simulink model "hexAddFm"  (R2024a)
settings: configuration reference "standardSILConfiguraitonParams" (kept outside this file)
settings Model: Creator=GTAR  LastModifiedBy=jerem
settings ConfigSetRef: SourceName=standardSILConfiguraitonParams  SourceLocation=Base Workspace

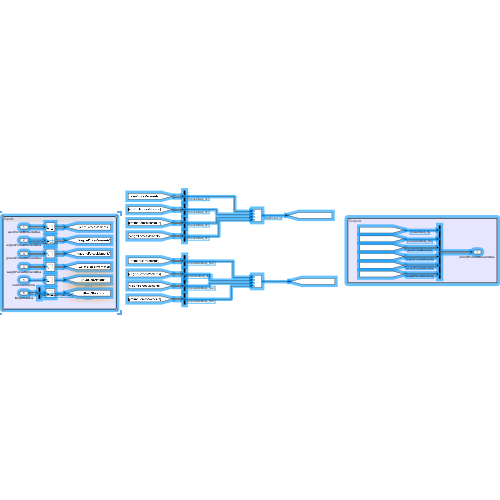
[thumbnail: Simulink's stored preview of the top-level diagram]
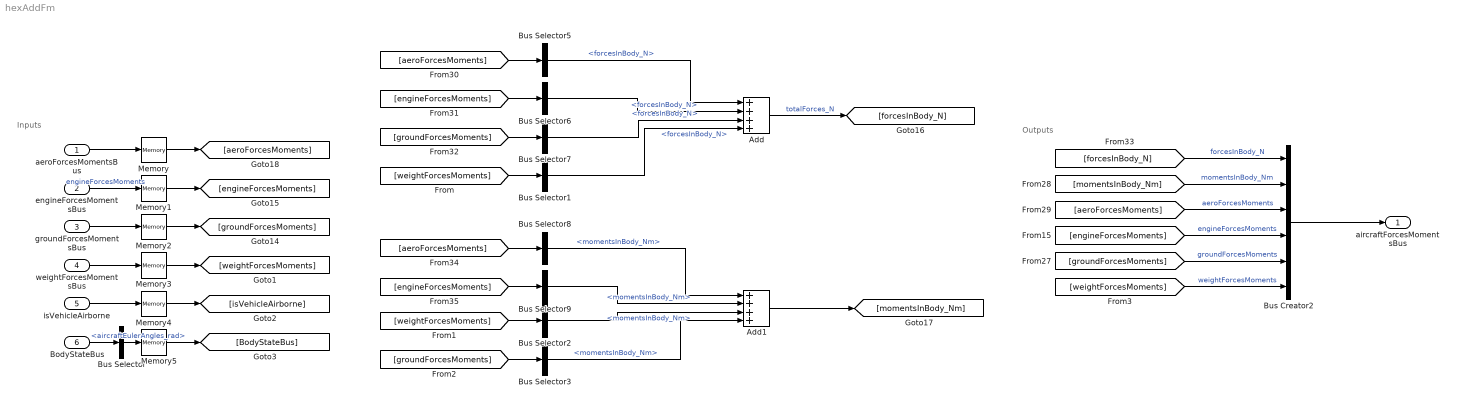
== system hexAddFm ==
  note: Outputs
  note: Inputs
  aeroForcesMomentsBus : Inport  OutDataTypeStr=Bus: ComponentForcesMomentsBus  SampleTime=0
  engineForcesMomentsBus : Inport  Port=2  OutDataTypeStr=Bus: ComponentForcesMomentsBus
  groundForcesMomentsBus : Inport  Port=3  OutDataTypeStr=Bus: ComponentForcesMomentsBus  SampleTime=0
  weightForcesMomentsBus : Inport  Port=4  OutDataTypeStr=Bus: ComponentForcesMomentsBus  SampleTime=0
  isVehicleAirborne : Inport  Port=5  OutDataTypeStr=boolean
  BodyStateBus : Inport  Port=6  OutDataTypeStr=Bus: BodyStateBus  SampleTime=0  BusOutputAsStruct=on
  Add : Sum  Inputs=++++
  Add1 : Sum  Inputs=++++
  Bus Creator2 : BusCreator  Inputs=6  OutDataTypeStr=Bus: AircraftForcesMomentsBus
  Bus Selector : BusSelector  OutputSignals=aircraftEulerAngles_rad
  Bus Selector{1,5..7} (4 alike) : BusSelector  OutputSignals=forcesInBody_N
  Bus Selector{2..3,8..9} (4 alike) : BusSelector  OutputSignals=momentsInBody_Nm
  Memory{,1..5} (6 alike) : Memory
  aircraftForcesMomentsBus : Outport  OutDataTypeStr=Bus: AircraftForcesMomentsBus  SampleTime=0
  wires:
  Bus Selector3/1 -> Add1/4  "<momentsInBody_Nm>"
  [groundForcesMoments] -> Bus Selector3/1
  Add1/1 -> [momentsInBody_Nm]
  Bus Selector6/1 -> Add/2  "<forcesInBody_N>"
  Memory5/1 -> [BodyStateBus]
  Bus Selector/1 -> Memory5/1  "<aircraftEulerAngles_rad>"
  Memory4/1 -> [isVehicleAirborne]
  [weightForcesMoments] -> Bus Selector2/1
  [groundForcesMoments] -> Bus Selector7/1
  BodyStateBus/1 -> Bus Selector/1
  [engineForcesMoments] -> Bus Selector9/1
  Bus Selector1/1 -> Add/4  "<forcesInBody_N>"
  [weightForcesMoments] -> Bus Selector1/1
  [momentsInBody_Nm] -> Bus Creator2/2  "momentsInBody_Nm"
  Bus Selector2/1 -> Add1/3  "<momentsInBody_Nm>"
  isVehicleAirborne/1 -> Memory4/1
  Memory2/1 -> [groundForcesMoments]
  Bus Creator2/1 -> aircraftForcesMomentsBus/1
  Memory3/1 -> [weightForcesMoments]
  Bus Selector5/1 -> Add/1  "<forcesInBody_N>"
  [weightForcesMoments] -> Bus Creator2/6  "weightForcesMoments"
  [groundForcesMoments] -> Bus Creator2/5  "groundForcesMoments"
  aeroForcesMomentsBus/1 -> Memory/1
  [engineForcesMoments] -> Bus Selector6/1
  Add/1 -> [forcesInBody_N]  "totalForces_N"
  [aeroForcesMoments] -> Bus Creator2/3  "aeroForcesMoments"
  groundForcesMomentsBus/1 -> Memory2/1
  Memory/1 -> [aeroForcesMoments]
  Bus Selector8/1 -> Add1/1  "<momentsInBody_Nm>"
  engineForcesMomentsBus/1 -> Memory1/1  "engineForcesMoments"
  [aeroForcesMoments] -> Bus Selector8/1
  Bus Selector9/1 -> Add1/2  "<momentsInBody_Nm>"
  [engineForcesMoments] -> Bus Creator2/4  "engineForcesMoments"
  Bus Selector7/1 -> Add/3  "<forcesInBody_N>"
  Memory1/1 -> [engineForcesMoments]
  [aeroForcesMoments] -> Bus Selector5/1
  [forcesInBody_N] -> Bus Creator2/1  "forcesInBody_N"
  weightForcesMomentsBus/1 -> Memory3/1
